simulink model "Boeing787_debug"  (R2015b)
settings: Solver=ode23tb  SolverMode=SingleTasking  StartTime=0.0  StopTime=18000  RelTol=1e-3
InitFcn:
  | load('SampleOutput.mat')
  | 
  | load('SampleFuelBurn.mat')
StartFcn:
  | tic
StopFcn:
  | ttt = toc
  | tend = eval(get_param(bdroot,'StopTime'));
  | disp(['Total Simulation Time (s) = ' num2str(ttt) 's']);
  | RTR =  ttt/tend
  | disp(['Simulation Speed is ' num2str(tend/ttt) 'x faster than real-time']);
values from neighbouring files (symbols this model uses):
  CurrentMission = Mission(i)    [mission_plan.m]
undefined symbols (not defined in the file or in its folder): FuelBurn, seed
libraries: PowerFlowLib x20, simulink x12, powerlib_meascontrol x1
(part 1 of 17)
settings Model: Creator=Bradford  LastModifiedBy=mwillms4
settings DataIOCC: SaveFormat=Array  SignalLoggingSaveFormat=ModelDataLogs
settings OptimizationCC: BlockReduction=off  BooleanDataType=off
settings DebuggingCC: SaveWithParameterizedLinksMsg=none  UnderspecifiedInitializationDetection=Classic  MergeDetectMultiDrivingBlocksExec=none  SignalResolutionControl=TryResolveAllWithWarning  MultiTaskDSMMsg=warning  MultiTaskCondExecSysMsg=none  StateNameClashWarn=warning
settings HardwareCC: ProdBitPerPointer=32  ProdLargestAtomicFloat=None  ProdIntDivRoundTo=Undefined  ProdEndianess=Unspecified  ProdWordSize=32  ProdHWDeviceType=32-bit Generic  TargetUnknown=on
settings GRTTargetCC: GeneratePreprocessorConditionals=Disable all
settings ConfigComp: CovModelRefEnable=Off

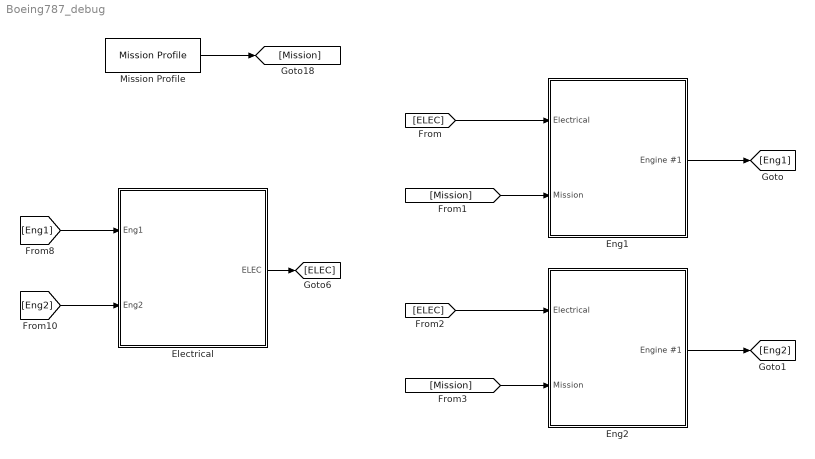
== system Boeing787_debug ==
  Electrical : Subsystem
  Eng1 : Subsystem
  Eng2 : Subsystem
  Mission Profile : PowerFlowLib/Mission Profile/Mission Profile  mssn_check=off  mssn_prof=MSSN  del_P=0  del_T=0  del_rho=0  pres_msl=101.3  temp_msl=15  dens_msl=1.229
  wires:
  [ELEC] -> Eng1/1(Electrical)
  [Mission] -> Eng1/2(Mission)
  Eng1/1(Engine #1) -> [Eng1]
  [Eng1] -> Electrical/1(Eng1)
  Mission Profile/1 -> [Mission]
  [Eng2] -> Electrical/2(Eng2)
  Electrical/1(ELEC) -> [ELEC]
  [ELEC] -> Eng2/1(Electrical)
  [Mission] -> Eng2/2(Mission)
  Eng2/1(Engine #1) -> [Eng2]
